simulink model "rct_ulinearize_builtin"  (R2023a)
settings: Solver=ode45  StartTime=0  StopTime=10  RelTol=1e-3  EnableMultiTasking=on
model workspace (MAT data in the model file):
  PrivateRobust.SpecifiedUncertainValues = struct([])
  PrivateRobust.UncertainValues.aa = 1.07418054116
  PrivateRobust.UncertainValues.a = -5.46136545551
  PrivateRobust.ArrayUncertainValues{1}.a = -5.56208162734
  PrivateRobust.ArrayUncertainValues{2} = struct([])
  PrivateRobust.ArrayUncertainValues{3}.a = -5.90591076757
  PrivateRobust.ArrayUncertainValues{4}.a = -4.64227056626
  PrivateRobust.ArrayUncertainValues{5}.a = -4.64140718833
  PrivateRobust.ArrayUncertainValues{6}.aa = 1.08987326037
  PrivateRobust.ArrayUncertainValues{6}.a = -5.23299584502
  PrivateRobust.ArrayUncertainValues{7}.aa = 1.00511153425
  PrivateRobust.ArrayUncertainValues{7}.a = -4.33806930778
  PrivateRobust.ArrayUncertainValues{8}.aa = 0.820050092309
  PrivateRobust.ArrayUncertainValues{8}.a = -5.89307672991
  PrivateRobust.ArrayUncertainValues{9}.aa = 1.00776627825
  PrivateRobust.ArrayUncertainValues{9}.a = -4.65770123185
  PrivateRobust.ArrayUncertainValues{10}.aa = 0.804583626119
  PrivateRobust.ArrayUncertainValues{10}.a = -5.23316869849
  PrivateRobust.ArrayUncertainValues{11}.aa = 0.837592570954
  PrivateRobust.ArrayUncertainValues{11}.a = -5.16502805108
  PrivateRobust.ArrayUncertainValues{12}.aa = 1.04429113917
  PrivateRobust.ArrayUncertainValues{12}.a = -4.82204671429
  PrivateRobust.ArrayUncertainValues{13}.aa = 1.08918946485
  PrivateRobust.ArrayUncertainValues{13}.a = -4.30766621898
  PrivateRobust.ArrayUncertainValues{14}.aa = 1.00705436376
  PrivateRobust.ArrayUncertainValues{14}.a = -5.81607021848
  PrivateRobust.ArrayUncertainValues{15}.aa = 1.03722527302
  PrivateRobust.ArrayUncertainValues{15}.a = -5.1680012863
  PrivateRobust.ArrayUncertainValues{16}.aa = 1.04730583277
  PrivateRobust.ArrayUncertainValues{16}.a = -4.17935833902
  PrivateRobust.ArrayUncertainValues{17}.aa = 1.05951613469
  PrivateRobust.ArrayUncertainValues{17}.a = -5.47509401267
  PrivateRobust.ArrayUncertainValues{18}.aa = 0.827188232014
  PrivateRobust.ArrayUncertainValues{18}.a = -4.52783623083
  PrivateRobust.ArrayUncertainValues{19}.aa = 0.948272444576
  PrivateRobust.ArrayUncertainValues{19}.a = -4.73472286422
  PrivateRobust.ArrayUncertainValues{20}.aa = 1.05839420523
  PrivateRobust.ArrayUncertainValues{20}.a = -4.01792522893
  PrivateRobust.ArrayUncertainValues{21}.aa = 0.960548592913
  PrivateRobust.ArrayUncertainValues{21}.a = -5.5059222288
  PrivateRobust.ArrayUncertainValues{22}.aa = 1.09735950499
  PrivateRobust.ArrayUncertainValues{22}.a = -4.55467919845
  PrivateRobust.ArrayUncertainValues{23}.aa = 1.05779906849
  PrivateRobust.ArrayUncertainValues{23}.a = -4.69696285049
  PrivateRobust.ArrayUncertainValues{24}.aa = 0.84065638456
  PrivateRobust.ArrayUncertainValues{24}.a = -4.7367305638
  PrivateRobust.ArrayUncertainValues{25}.aa = 1.08164815058
  PrivateRobust.ArrayUncertainValues{25}.a = -5.45458006647
  PrivateRobust.ArrayUncertainValues{26}.aa = 0.982292372757
  PrivateRobust.ArrayUncertainValues{26}.a = -4.46701044425
  PrivateRobust.ArrayUncertainValues{27}.aa = 0.99397232014
  PrivateRobust.ArrayUncertainValues{27}.a = -5.52445113264
  PrivateRobust.ArrayUncertainValues{28}.aa = 0.929377377992
  PrivateRobust.ArrayUncertainValues{28}.a = -5.28147004139
  PrivateRobust.ArrayUncertainValues{29}.aa = 0.885643980778
  PrivateRobust.ArrayUncertainValues{29}.a = -5.02696523398
  PrivateRobust.ArrayUncertainValues{30}.aa = 1.08382050835
  PrivateRobust.ArrayUncertainValues{30}.a = -4.18158379671
  PrivateRobust.ArrayUncertainValues{31}.aa = 0.834263453507
  PrivateRobust.ArrayUncertainValues{31}.a = -4.19069381533
  PrivateRobust.ArrayUncertainValues{32}.aa = 1.00120247947
  PrivateRobust.ArrayUncertainValues{32}.a = -4.96741607271
  PrivateRobust.ArrayUncertainValues{33}.aa = 0.945121292065
  PrivateRobust.ArrayUncertainValues{33}.a = -4.02671577596
  PrivateRobust.ArrayUncertainValues{34}.aa = 0.998387306823
  PrivateRobust.ArrayUncertainValues{34}.a = -5.46771098555
  PrivateRobust.ArrayUncertainValues{35}.aa = 0.849911153486
  PrivateRobust.ArrayUncertainValues{35}.a = -4.10447150008
  PrivateRobust.ArrayUncertainValues{36}.aa = 0.84121022886
  PrivateRobust.ArrayUncertainValues{36}.a = -4.99858581042
  PrivateRobust.ArrayUncertainValues{37}.aa = 0.966518510503
  PrivateRobust.ArrayUncertainValues{37}.a = -5.44583639942
  PrivateRobust.ArrayUncertainValues{38}.aa = 1.08649047352
  PrivateRobust.ArrayUncertainValues{38}.a = -4.94050521261
  PrivateRobust.ArrayUncertainValues{39}.aa = 0.990288701858
  PrivateRobust.ArrayUncertainValues{39}.a = -4.11804009234
  PrivateRobust.ArrayUncertainValues{40}.aa = 0.828617130338
  PrivateRobust.ArrayUncertainValues{40}.a = -4.47697147563
  PrivateRobust.ArrayUncertainValues{41}.aa = 1.06105611857
  PrivateRobust.ArrayUncertainValues{41}.a = -4.34436539949
  PrivateRobust.ArrayUncertainValues{42}.aa = 0.866839825527
  PrivateRobust.ArrayUncertainValues{42}.a = -5.96826459745
  PrivateRobust.ArrayUncertainValues{43}.aa = 1.04464561213
  PrivateRobust.ArrayUncertainValues{43}.a = -4.26350573649
  PrivateRobust.ArrayUncertainValues{44}.aa = 1.03179870299
  PrivateRobust.ArrayUncertainValues{44}.a = -4.52755097138
  PrivateRobust.ArrayUncertainValues{45}.aa = 1.05225696788
  PrivateRobust.ArrayUncertainValues{45}.a = -4.00108424202
  PrivateRobust.ArrayUncertainValues{46}.aa = 1.08229967821
  PrivateRobust.ArrayUncertainValues{46}.a = -5.53361024313
  PrivateRobust.ArrayUncertainValues{47}.aa = 0.940695113779
  PrivateRobust.ArrayUncertainValues{47}.a = -5.29796950393
  PrivateRobust.ArrayUncertainValues{48}.aa = 1.00350860581
  PrivateRobust.ArrayUncertainValues{48}.a = -4.81777283494
  PrivateRobust.ArrayUncertainValues{49}.aa = 1.07496966765
  PrivateRobust.ArrayUncertainValues{49}.a = -5.1758384589
  PrivateRobust.ArrayUncertainValues{50}.aa = 1.07418054116
  PrivateRobust.ArrayUncertainValues{50}.a = -5.46136545551
  PrivateRobust.AlreadyUsed = 1
  PrivateRobust.CheckUConsistent = 0
  PrivateRobust.UssBlockAtomCell = struct([])
  PrivateRobust.Seed = 2097586808
  PrivateRobust.SeedN = 931316785
libraries: slpidlib x1
settings Model: Creator=The MathWorks, Inc.  LastModifiedBy=The MathWorks, Inc.
settings SolverCC: AlgebraicLoopSolver=TrustRegion  MaxZcPerStep=1
settings DataIOCC: LimitDataPoints=on  SaveFormat=Array  ReturnWorkspaceOutputs=off
settings OptimizationCC: DefaultParameterBehavior=Inlined  BufferReuse=off  ExpressionDepthLimit=2147483647  InitFltsAndDblsToZero=on  LifeSpan=inf
settings DebuggingCC: SaveWithParameterizedLinksMsg=none  UnderspecifiedInitializationDetection=Classic  MergeDetectMultiDrivingBlocksExec=none  SignalResolutionControl=TryResolveAllWithWarning  MultiTaskDSMMsg=warning  MultiTaskCondExecSysMsg=none  FcnCallInpInsideContextMsg=warning  UnconnectedInputMsg=warning  UnconnectedOutputMsg=warning  UnconnectedLineMsg=warning  StateNameClashWarn=warning  SFUnexpectedBacktrackingDiag=warning  SFNoUnconditionalDefaultTransitionDiag=warning  SFExecutionAtInitializationDiag=none  ArithmeticOperatorsInVariantConditions=warning
settings HardwareCC: ProdBitPerPointer=32  ProdBitPerSizeT=32  ProdBitPerPtrDiffT=32  ProdLargestAtomicFloat=None  ProdIntDivRoundTo=Undefined  ProdEndianess=Unspecified  ProdWordSize=32  ProdHWDeviceType=32-bit Generic
settings ModelReferenceCC: EnableRefExpFcnMdlSchedulingChecks=on  PropagateSignalLabelsOutOfModel=off
settings SFSimCC: SimUseLocalCustomCode=off  CustomCodeUndefinedFunction=UseInterfaceOnly
settings RTWCC: RTWUseLocalCustomCode=off  DLArmComputeVersion=19.05
settings CodeAppCC: StateflowObjectComments=on
settings GRTTargetCC: TargetFcnLib=ansi_tfl_tmw.mat  TargetLangStandard=C89/C90 (ANSI)  CombineOutputUpdateFcns=off  GRTInterface=on
settings ConfigComp: CovMetricSettings=dw  CovSaveCumulativeToWorkspaceVar=on  CovSaveSingleToWorkspaceVar=on  CovExternalEMLEnable=off  CovSFcnEnable=off

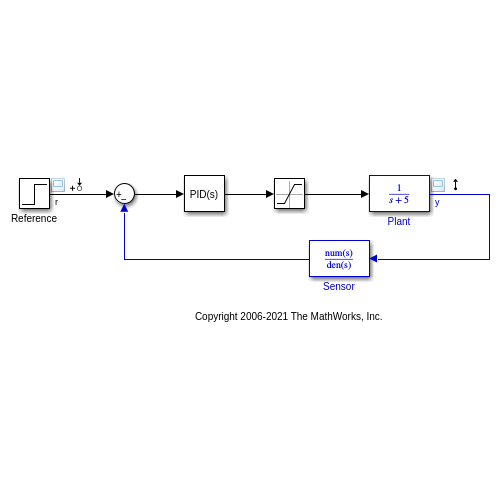
[thumbnail: Simulink's stored preview of the top-level diagram]
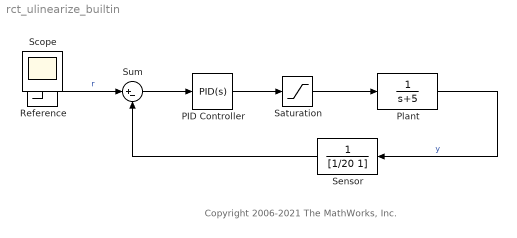
== system rct_ulinearize_builtin ==
  note: Copyright 2006-2021 The MathWorks, Inc.
  PID Controller : slpidlib/PID Controller  Tag=PID1  Controller=PID  Form=Parallel  TimeDomain=Continuous-time  UseExternalTs=off  SampleTime=1  IntegratorMethod=Forward Euler  FilterMethod=Forward Euler  ControllerParametersSource=internal  P=0.138669  I=3.904337  UseKiTs=off  D=-0.019669  N=6.838200  UseFilter=on  TunerSelectOption=Transfer Function Based (PID Tuner App)  ZeroCross=off  InitialConditionSource=internal  InitialConditionForIntegrator=0  InitialConditionForFilter=0  DifferentiatorICPrevScaledInput=0  ExternalReset=none  TrackingMode=off  Kt=1  LimitOutput=off  SatLimitsSource=internal  UpperSaturationLimit=inf  LowerSaturationLimit=-inf  LinearizeAsGain=off  AntiWindupMode=none  Kb=1  LimitIntegrator=off  UpperIntegratorSaturationLimit=inf  LowerIntegratorSaturationLimit=-inf  POutMin=[ ]  POutMax=[ ]  IOutMin=[ ]  IOutMax=[ ]  DOutMin=[ ]  DOutMax=[ ]  NOutMin=[ ]  NOutMax=[ ]  SumOutMin=[ ]  SumOutMax=[ ]  SaturationOutMin=[ ]  SaturationOutMax=[ ]  PParamMin=[ ]  PParamMax=[ ]  IParamMin=[ ]  IParamMax=[ ]  DParamMin=[ ]  DParamMax=[ ]  NParamMin=[ ]  NParamMax=[ ]  KbParamMin=[ ]  KbParamMax=[ ]  KtParamMin=[ ]  KtParamMax=[ ]  KbOutMin=[ ]  KbOutMax=[ ]  KtOutMin=[ ]  KtOutMax=[ ]  IntegratorOutMin=[ ]  IntegratorOutMax=[ ]  FilterOutMin=[ ]  FilterOutMax=[ ]  SumI1OutMin=[ ]  SumI1OutMax=[ ]  SumI2OutMin=[ ]  SumI2OutMax=[ ]  SumI3OutMin=[ ]  SumI3OutMax=[ ]  SumI4OutMin=[]  SumI4OutMax=[]  SumDOutMin=[ ]  SumDOutMax=[ ]  DifferentiatorOutMin=[]  DifferentiatorOutMax=[]  FilterDiffOutCoefMin=[]  FilterDiffOutCoefMax=[]  ReciprocalOutMin=[]  ReciprocalOutMax=[]  SumDenOutMin=[]  SumDenOutMax=[]  SumNumOutMin=[]  SumNumOutMax=[]  DivideOutMin=[]  DivideOutMax=[]  UdiffTsProdOutMin=[]  UdiffTsProdOutMax=[]  NTsProdOutMin=[]  NTsProdOutMax=[]  UintegralTsProdOutMin=[]  UintegralTsProdOutMax=[]  UngainTsProdOutMin=[]  UngainTsProdOutMax=[]  ClampingZeroOutDataTypeStr=Inherit: Inherit via back propagation  ClampingZeroOutMin=[]  ClampingZeroOutMax=[]  FilterDenConstantOutDataTypeStr=Inherit: Inherit via back propagation  FilterDenConstantOutMin=[]  FilterDenConstantOutMax=[]  PCopyOutDataTypeStr=Inherit: Inherit via back propagation  PCopyOutMin=[]  PCopyOutMax=[]  NCopyOutDataTypeStr=Inherit: Inherit via back propagation  NCopyOutMin=[]  NCopyOutMax=[]  IntegratorContinuousStateAttributes=''  IntegratorStateMustResolveToSignalObject=off  IntegratorRTWStateStorageClass=Auto  FilterContinuousStateAttributes=''  FilterStateMustResolveToSignalObject=off  FilterRTWStateStorageClass=Auto  ParallelPVariant=InternalParameters  IdealPVariant=Disabled  IVariant=InternalParameters  DVariant=InternalParameters  IntegratorVariant=Continuous  SatVariant=Disabled  AWVariant=Passthrough  PCopyVariant=Disabled  TRVariant=Disabled  FdbkBlocksVariant=Forward  IdealPFdbkVariant=Disabled  SatFdbkVariant=Disabled  DerivativeFilterVariant=ContFilter  NVariant=InternalParameters  NCopyVariant=Disabled  FilterICVariant=InternalICsFilter  IntegratorICVariant=InternalICs  ExternalResetVariant=Disabled  TRSumVariant=Passthrough  SumFdbkVariant=Disabled  SumVariant=Sum_PID  TsampFilterVariant=InternalTs  TsampNgainVariant=Passthrough  TsampIntegralVariant=Disabled_SignalSpec  ExternalSaturationOutDataTypeStr=Inherit: Same as second input
  Plant : TransferFcn  SCDEnableBlockLinearizationSpecification=on  Denominator=[1 5]
  Reference : Step  SampleTime=0
  Saturation : Saturate  UpperLimit=1  LowerLimit=-1
  Sensor : TransferFcn  SCDEnableBlockLinearizationSpecification=on  Denominator=[1/20 1]
  Sum : Sum  Inputs=|+-
  Scope : Scope
  wires:
  Sensor/1 -> Sum/2
  Reference/1 -> Sum/1  "r"
  Plant/1 -> Sensor/1  "y"
  PID Controller/1 -> Saturation/1
  Sum/1 -> PID Controller/1
  Saturation/1 -> Plant/1
